simulink model "simulation"  (R2023b)
settings: Solver=VariableStepAuto  StartTime=0.0  StopTime=1.2  RelTol=1e-3
values from neighbouring files (symbols this model uses):
  J = [0 -1; 1 0]    [SafetyFilterSystemDPC.m]    (also in init.m)
undefined symbols (not defined in the file or in its folder): ctrl, DiscIntNeverNeededParam, fdesignblkfcn, gcbh, grid, infinite_bus, load1, overcurr_ctrl, pll, pq_ctrl, pv, sim, soa
libraries: spsabctodq0Lib x8, eeGeneralControl x6, spsControlledVoltageSourceLib x6, eeDiscretePi x5, dsparch4 x4, spsBreakerLib x3, spsThreePhaseSeriesRLCBranchLib x3, spsdq0toabcLib x2, spsThreePhaseBreakerLib x2, simulink x1, spsGroundLib x1, spsThreePhaseVIMeasurementLib x1
settings Model: SimulationMode=accelerator  Creator=ma1155716  LastModifiedBy=ma1155716

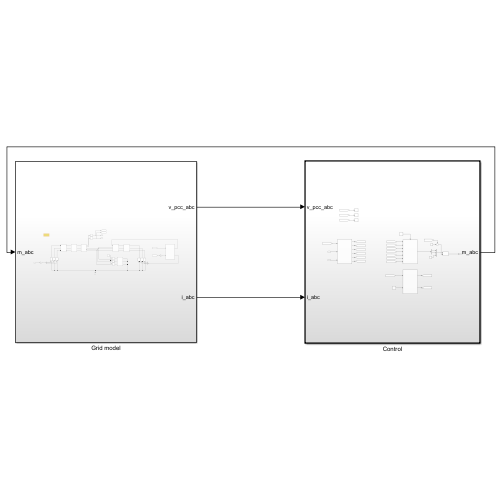
[thumbnail: Simulink's stored preview of the top-level diagram]
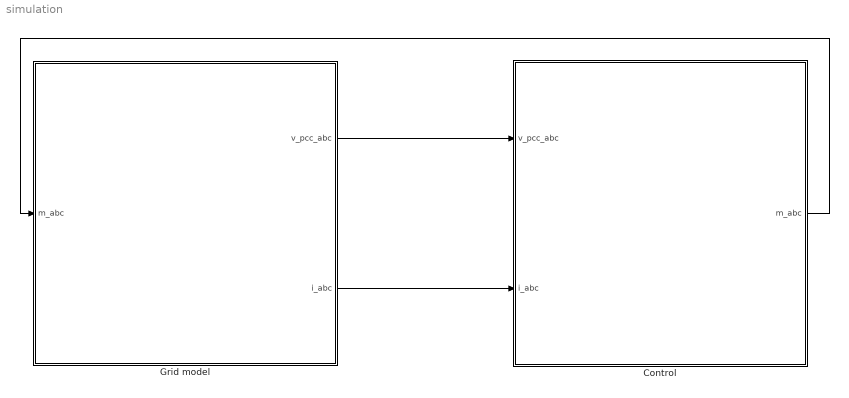
== system simulation ==
  Control : Subsystem  TreatAsAtomicUnit=on
  Grid model : Subsystem
  wires:
  Grid model/1(v_pcc_abc) -> Control/1(v_pcc_abc)
  Control/1(m_abc) -> Grid model/1(m_abc)
  Grid model/2(i_abc) -> Control/2(i_abc)

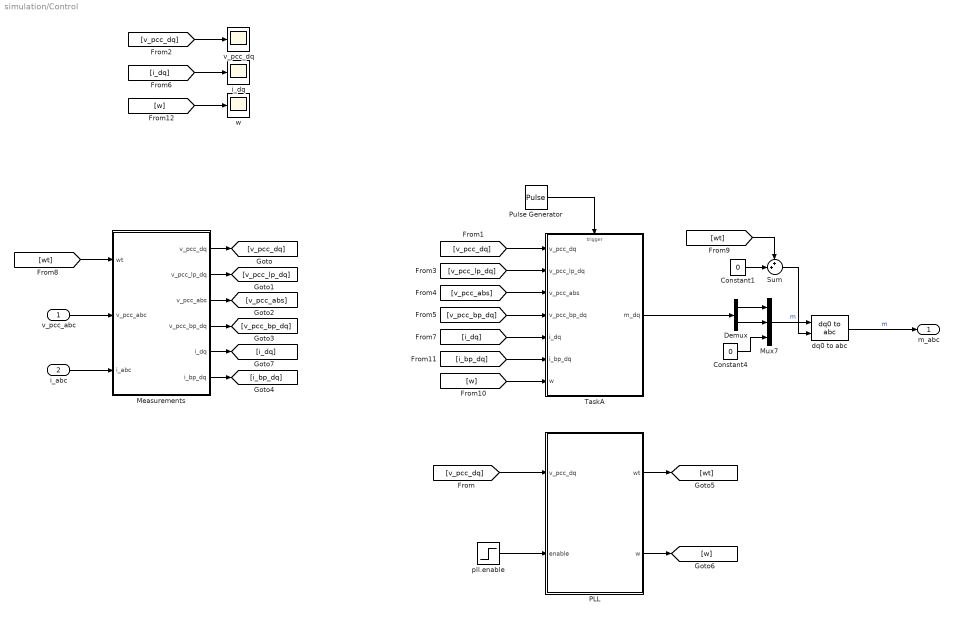
== system simulation/Control ==
  v_pcc_abc : Inport
  i_abc : Inport  Port=2
  Constant1 : Constant  Value=0
  Constant4 : Constant  Value=0
  Demux : Demux  Outputs=2
  Measurements : Subsystem
  Mux7 : Mux  Inputs=3
  PLL : Subsystem
  Pulse Generator : DiscretePulseGenerator  PulseType=Time based  Period=ctrl.ts  PulseWidth=50
  Sum : Sum  Inputs=++|
  TaskA : Subsystem
  dq0 to abc : spsdq0toabcLib/dq0 to abc  Alignment=Aligned with phase A axis
  i_dq : Scope
  "pll.enable " : Step  Time=pll.enable
  v_pcc_dq : Scope
  w : Scope
  m_abc : Outport  InitialOutput=[1;0;0]
  wires:
  v_pcc_abc/1 -> Measurements/2(v_pcc_abc)
  i_abc/1 -> Measurements/3(i_abc)
  Pulse Generator/1 -> TaskA/Trigger
  Demux/1 -> Mux7/1
  Constant4/1 -> Mux7/3
  Demux/2 -> Mux7/2
  TaskA/1(m_dq) -> Demux/1
  Mux7/1 -> dq0 to abc/1  "m"
  dq0 to abc/1 -> m_abc/1  "m"
  Sum/1 -> dq0 to abc/2
  Constant1/1 -> Sum/2
  Measurements/1(v_pcc_dq) -> [v_pcc_dq]
  [v_pcc_dq] -> PLL/1(v_pcc_dq)
  [v_pcc_dq] -> TaskA/1(v_pcc_dq)
  Measurements/2(v_pcc_lp_dq) -> [v_pcc_lp_dq]
  [v_pcc_lp_dq] -> TaskA/2(v_pcc_lp_dq)
  [v_pcc_dq] -> v_pcc_dq/1
  Measurements/3(v_pcc_abs) -> [v_pcc_abs]
  Measurements/4(v_pcc_bp_dq) -> [v_pcc_bp_dq]
  [v_pcc_abs] -> TaskA/3(v_pcc_abs)
  [v_pcc_bp_dq] -> TaskA/4(v_pcc_bp_dq)
  Measurements/6(i_bp_dq) -> [i_bp_dq]
  [i_dq] -> i_dq/1
  [i_dq] -> TaskA/5(i_dq)
  PLL/1(wt) -> [wt]
  [wt] -> Measurements/1(wt)
  [wt] -> Sum/1
  PLL/2(w) -> [w]
  [w] -> TaskA/7(w)
  Measurements/5(i_dq) -> [i_dq]
  [i_bp_dq] -> TaskA/6(i_bp_dq)
  "pll.enable "/1 -> PLL/2(enable)
  [w] -> w/1

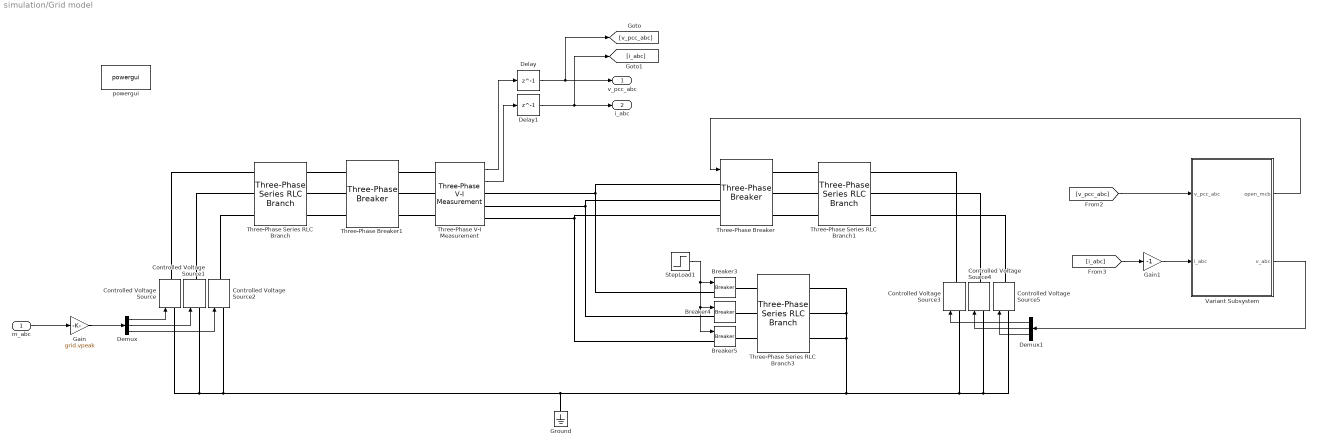
== system simulation/Grid model ==
  m_abc : Inport
  Breaker3 : spsBreakerLib/Breaker  InitialState=0  SwitchingTimes="[1/60  5/60]"  External=on  BreakerResistance=0.01  SnubberResistance=1e6  SnubberCapacitance=inf  Measurements=None  MoreParameters=on  NoBreakLoop=off
  Breaker4 : spsBreakerLib/Breaker  InitialState=0  SwitchingTimes="[1/60  5/60]"  External=on  BreakerResistance=0.01  SnubberResistance=1e6  SnubberCapacitance=inf  Measurements=None  MoreParameters=on  NoBreakLoop=off
  Breaker5 : spsBreakerLib/Breaker  InitialState=0  SwitchingTimes="[1/60  5/60]"  External=on  BreakerResistance=0.01  SnubberResistance=1e6  SnubberCapacitance=inf  Measurements=None  MoreParameters=on  NoBreakLoop=off
  Controlled Voltage Source{,1..5} (6 alike) : spsControlledVoltageSourceLib/Controlled Voltage Source  Initialize=on  Source_Type=AC  Amplitude=0  Phase=0  Frequency=0  Measurements=None
  Delay : Delay  DelayLength=1  InitialCondition=0  SampleTime=sim.ts
  Delay1 : Delay  DelayLength=1  InitialCondition=0  SampleTime=sim.ts
  Demux : Demux  Outputs=3
  Demux1 : Demux  Outputs=3
  Gain : Gain  Gain=grid.vpeak
  Gain1 : Gain  Gain=-1
  Ground : spsGroundLib/Ground  LConnTagsString=a
  StepLoad1 : Step  Time=load1.stepTime  SampleTime=0
  Three-Phase Series RLC Branch : spsThreePhaseSeriesRLCBranchLib/Three-Phase Series RLC Branch  LConnTagsString=A|B|C  RConnTagsString=A|B|C  BranchType=RL  Resistance=grid.r1_si  Inductance=grid.l1_si  Capacitance=1e-6  Measurements=None
  Three-Phase Series RLC Branch1 : spsThreePhaseSeriesRLCBranchLib/Three-Phase Series RLC Branch  LConnTagsString=A|B|C  RConnTagsString=A|B|C  BranchType=RL  Resistance=grid.r2_si  Inductance=grid.l2_si  Capacitance=1e-6  Measurements=None
  Three-Phase Series RLC Branch3 : spsThreePhaseSeriesRLCBranchLib/Three-Phase Series RLC Branch  LConnTagsString=A|B|C  RConnTagsString=A|B|C  BranchType=RL  Resistance=load1.r_si  Inductance=load1.l_si  Capacitance=1e-6  Measurements=None
  Three-Phase V-I Measurement : spsThreePhaseVIMeasurementLib/Three-Phase V-I Measurement  VoltageMeasurement=phase-to-ground  SetLabelV=off  LabelV=Vabc  Vpu=off  VpuLL=off  CurrentMeasurement=yes  SetLabelI=off  LabelI=Iabc  Ipu=off  Pbase=100e6  Vbase=500e3  OutputType=Complex  PhasorSimulation=off  PSBequivalent=0
  Three-Phase Breaker : spsThreePhaseBreakerLib/Three-Phase Breaker  InitialState=open  SwitchA=on  SwitchB=on  SwitchC=on  SwitchTimes=[grid.close_mcb2]  External=on  BreakerResistance=0.01  SnubberResistance=1e6  SnubberCapacitance=inf  Measurements=None
  Three-Phase Breaker1 : spsThreePhaseBreakerLib/Three-Phase Breaker  InitialState=open  SwitchA=on  SwitchB=on  SwitchC=on  SwitchTimes=[0]  External=off  BreakerResistance=0.01  SnubberResistance=1e6  SnubberCapacitance=inf  Measurements=None
  Variant Subsystem : Subsystem  Variant=on
  powergui : spspowerguiLib/powergui  Priority=1  SimulationMode=Discrete  SampleTime=sim.ts  frequency=60  Iterations=50  frequencyindice=0  Pbase=100e6  ErrMax=1e-4  UnitsV=kV  UnitsW=MW  buscounter=0  FunctionMessages=off  echomessages=off  EnableUseOfTLC=off  CurrentSourceSwitches=off  DisableSnubberDevices=off  DisableRonSwitches=off  DisableVfSwitches=off  DisplayEquations=off  AutomaticDiscreteSolvers=off  SolverType=Tustin/Backward Euler (TBE)  Interpol=off  ExternalGateDelay=off  methode=off  Ts=100  x0status=blocks  SPID=on  SwTol=0  HookPort=off  NonlinearTolerance=1e-4  nMaxIteration=100  ContinueOnMaxIteration=off  RestoreLinks=warning  ResistiveCurrentMeasurement=off  Frange=[0:2:500]  Ylog=off  Xlog=on  ShowGrid=off  save=off  variable=ZData  structure=0  ZoomFFT=off  StartTime=0.0  cycles=1  DisplayStyle=1  fundamental=60  FreqAxis=off  MaxFrequency=1000  frequencyindicesteady=1  RmsSteady=1  display=off
  v_pcc_abc : Outport
  i_abc : Outport  Port=2
  wires:
  m_abc/1 -> Gain/1
  Demux/1 -> Controlled Voltage Source/1
  Demux/2 -> Controlled Voltage Source1/1
  Demux/3 -> Controlled Voltage Source2/1
  Demux1/3 -> Controlled Voltage Source5/1
  Demux1/1 -> Controlled Voltage Source3/1
  Three-Phase V-I Measurement/1 -> Delay/1
  Three-Phase V-I Measurement/2 -> Delay1/1
  Gain/1 -> Demux/1
  Demux1/2 -> Controlled Voltage Source4/1
  StepLoad1/1 -> Breaker5/1, Breaker4/1, Breaker3/1
  Delay1/1 -> [i_abc], i_abc/1
  Delay/1 -> [v_pcc_abc], v_pcc_abc/1
  [v_pcc_abc] -> Variant Subsystem/1(v_pcc_abc)
  [i_abc] -> Gain1/1
  Variant Subsystem/2(v_abc) -> Demux1/1
  Gain1/1 -> Variant Subsystem/2(i_abc)
  Variant Subsystem/1(open_mcb) -> Three-Phase Breaker/1
  connections:
  Three-Phase Series RLC Branch/LConn1 -- Controlled Voltage Source/RConn1
  Three-Phase Series RLC Branch/LConn2 -- Controlled Voltage Source1/RConn1
  Controlled Voltage Source2/RConn1 -- Three-Phase Series RLC Branch/LConn3
  Three-Phase Series RLC Branch/RConn1 -- Three-Phase Breaker1/LConn1
  Three-Phase Series RLC Branch/RConn2 -- Three-Phase Breaker1/LConn2
  Three-Phase Series RLC Branch/RConn3 -- Three-Phase Breaker1/LConn3
  Breaker3/LConn1 -- Three-Phase Breaker/LConn1 -- Three-Phase V-I Measurement/RConn1
  Breaker4/LConn1 -- Three-Phase V-I Measurement/RConn2 -- Three-Phase Breaker/LConn2
  Breaker5/LConn1 -- Three-Phase Breaker/LConn3 -- Three-Phase V-I Measurement/RConn3
  Controlled Voltage Source3/RConn1 -- Three-Phase Series RLC Branch1/RConn1
  Controlled Voltage Source4/RConn1 -- Three-Phase Series RLC Branch1/RConn2
  Controlled Voltage Source5/RConn1 -- Three-Phase Series RLC Branch1/RConn3
  Ground/LConn1 -- Controlled Voltage Source3/LConn1 -- Controlled Voltage Source5/LConn1 -- Controlled Voltage Source4/LConn1 -- Three-Phase Series RLC Branch3/RConn3 -- Three-Phase Series RLC Branch3/RConn2 -- Three-Phase Series RLC Branch3/RConn1 -- Controlled Voltage Source2/LConn1 -- Controlled Voltage Source1/LConn1 -- Controlled Voltage Source/LConn1
  Breaker4/RConn1 -- Three-Phase Series RLC Branch3/LConn2
  Breaker5/RConn1 -- Three-Phase Series RLC Branch3/LConn3
  Three-Phase Series RLC Branch3/LConn1 -- Breaker3/RConn1
  Three-Phase Series RLC Branch1/LConn1 -- Three-Phase Breaker/RConn1
  Three-Phase Series RLC Branch1/LConn2 -- Three-Phase Breaker/RConn2
  Three-Phase Series RLC Branch1/LConn3 -- Three-Phase Breaker/RConn3
  Three-Phase Breaker1/RConn1 -- Three-Phase V-I Measurement/LConn1
  Three-Phase Breaker1/RConn2 -- Three-Phase V-I Measurement/LConn2
  Three-Phase Breaker1/RConn3 -- Three-Phase V-I Measurement/LConn3

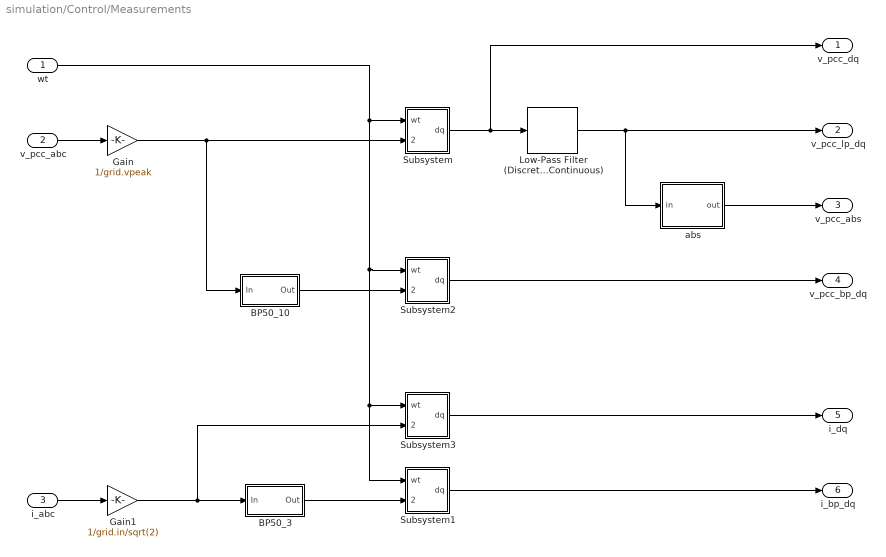
== system simulation/Control/Measurements ==
  wt : Inport
  v_pcc_abc : Inport  Port=2
  i_abc : Inport  Port=3
  BP50_10 : Subsystem  DialogController=fdesignblkfcn  InitFcn=fdesignblkfcn(gcbh, {'InitFcn'});  mask(Bandpass Filter){}
      mask help: dsp:DSPFilterDesignBlockDialog:BandpassFdesign_MaskDesc
      settings: CopyFcn=fdesignblkfcn(gcbh, {'CopyFcn'});
      mask Help: helpview(mapfilelocation('dsp'), 'dspbandpassfilter');
      mask Display: disp('Bandpass');
  BP50_3 : Subsystem  DialogController=fdesignblkfcn  InitFcn=fdesignblkfcn(gcbh, {'InitFcn'});  mask(Bandpass Filter){}
      mask help: dsp:DSPFilterDesignBlockDialog:BandpassFdesign_MaskDesc
      settings: CopyFcn=fdesignblkfcn(gcbh, {'CopyFcn'});
      mask Help: helpview(mapfilelocation('dsp'), 'dspbandpassfilter');
      mask Display: disp('Bandpass');
  Gain : Gain  Gain=1/grid.vpeak
  Gain1 : Gain  Gain=1/grid.in/sqrt(2)
  Low-Pass Filter (Discrete or Continuous) : eeGeneralControl/Low-Pass Filter (Discrete or Continuous)  K=1  T=1/grid.w0*10  B=inf  A=-inf  init_option=Inherited from block input  x0=0  Ts=-1
  Subsystem : Subsystem
  Subsystem1 : Subsystem
  Subsystem2 : Subsystem
  Subsystem3 : Subsystem
  abs : Subsystem
  v_pcc_dq : Outport
  v_pcc_lp_dq : Outport  Port=2
  v_pcc_abs : Outport  Port=3
  v_pcc_bp_dq : Outport  Port=4
  i_dq : Outport  Port=5
  i_bp_dq : Outport  Port=6
  wires:
  v_pcc_abc/1 -> Gain/1
  Subsystem/1(dq) -> v_pcc_dq/1, Low-Pass Filter (Discrete or Continuous)/1
  Gain/1 -> BP50_10/1(In), Subsystem/2(abc)
  i_abc/1 -> Gain1/1
  BP50_3/1(Out) -> Subsystem1/2(abc)
  Subsystem1/1(dq) -> i_bp_dq/1
  Gain1/1 -> Subsystem3/2(abc), BP50_3/1(In)
  Low-Pass Filter (Discrete or Continuous)/1 -> abs/1(in), v_pcc_lp_dq/1
  BP50_10/1(Out) -> Subsystem2/2(abc)
  Subsystem2/1(dq) -> v_pcc_bp_dq/1
  wt/1 -> Subsystem2/1(wt), Subsystem3/1(wt), Subsystem1/1(wt), Subsystem/1(wt)
  Subsystem3/1(dq) -> i_dq/1
  abs/1(out) -> v_pcc_abs/1

== system simulation/Control/PLL ==
  v_pcc_dq : Inport
  enable : Inport  Port=2
  Complex to Magnitude-Angle : ComplexToMagnitudeAngle
  Constant : Constant  Value=0
  Constant1 : Constant  Value=0
  Demux6 : Demux  Outputs=2
  Discrete PI Controller : eeDiscretePi/Discrete PI Controller  Kp=pll.kp  Ki=pll.ki  Kaw=1  x0=pll.init_w  Ts=-1
      settings: LibrarySourceBlock=ee_sl_lib/General Control/Discrete PI Controller
  Discrete-Time Integrator : DiscreteIntegrator  gainval=grid.w0  SampleTime=-1  ICPrevOutput=DiscIntNeverNeededParam  ICPrevScaledInput=DiscIntNeverNeededParam
  NOT1 : Logic  Operator=NOT  IconShape=distinctive  AllPortsSameDT=off  OutDataTypeStr=boolean
  Real-Imag to Complex : RealImagToComplex
  Switch : Switch  Criteria=u2 > Threshold  SaturateOnIntegerOverflow=off  InputSameDT=off
  Terminator7 : Terminator
  wt : Outport
  w : Outport  Port=2
  wires:
  v_pcc_dq/1 -> Demux6/1  "v_pcc_dq"
  Complex to Magnitude-Angle/1 -> Terminator7/1
  Demux6/2 -> Real-Imag to Complex/2  "v_pll_q"
  Complex to Magnitude-Angle/2 -> Switch/3  "theta_v_pll"
  Real-Imag to Complex/1 -> Complex to Magnitude-Angle/1
  Demux6/1 -> Real-Imag to Complex/1  "v_pll_d"
  Constant/1 -> Discrete PI Controller/2
  Discrete PI Controller/1 -> w/1, Discrete-Time Integrator/1
  Discrete-Time Integrator/1 -> wt/1
  NOT1/1 -> Switch/2, Discrete PI Controller/3
  enable/1 -> NOT1/1
  Switch/1 -> Discrete PI Controller/1
  Constant1/1 -> Switch/1

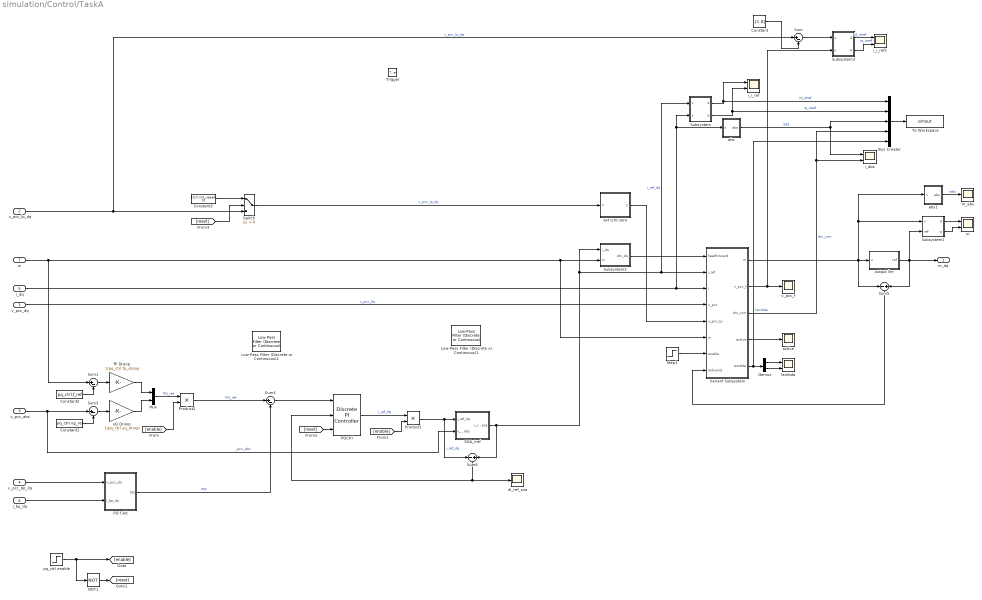
== system simulation/Control/TaskA ==
  v_pcc_dq : Inport
  v_pcc_lp_dq : Inport  Port=2
  v_pcc_abs : Inport  Port=3
  v_pcc_bp_dq : Inport  Port=4
  i_dq : Inport  Port=5
  i_bp_dq : Inport  Port=6
  w : Inport  Port=7
  Trigger : TriggerPort  VariantControl=(inherit)
  Bus Creator : BusCreator  Inputs=5
  Constant : Constant  Value=[1 0]
  Constant1 : Constant  Value=pq_ctrl.vg_ref
  Constant2 : Constant  Value=pq_ctrl.f_ref
  Constant3 : Constant  Value=[ctrl.init_vpeak; 0]
  Demux : Demux  Outputs=2
  Low-Pass Filter (Discrete or Continuous)1 : eeGeneralControl/Low-Pass Filter (Discrete or Continuous)  K=1  T=1e-3  B=inf  A=-inf  init_option=Inherited from block input  x0=0  Ts=-1
  Low-Pass Filter (Discrete or Continuous)2 : eeGeneralControl/Low-Pass Filter (Discrete or Continuous)  K=1  T=1e-2  B=inf  A=-inf  init_option=Inherited from block input  x0=0  Ts=-1
  Mux : Mux  Inputs=2
  NOT1 : Logic  Operator=NOT  IconShape=distinctive  AllPortsSameDT=off  OutDataTypeStr=boolean
  PQ Calc : Subsystem
  PQCtrl : eeDiscretePi/Discrete PI Controller  Kp=pq_ctrl.kp  Ki=pq_ctrl.ki  Kaw=100  x0=0  Ts=-1
      settings: LibrarySourceBlock=ee_sl_lib/General Control/Discrete PI Controller
  Product1 : Product
  Product2 : Product
  SOA_iref : Subsystem
  Step1 : Step  Time=overcurr_ctrl.enableTime
  Subsystem : Subsystem
  Subsystem1 : Subsystem
  Subsystem2 : Subsystem
  Subsystem3 : Subsystem
  Sum{,1,3..4} (4 alike) : Sum  Inputs=|+-
  Sum5 : Sum  Inputs=-|+
  Sum6 : Sum  Inputs=-|+
  Switch : Switch  Criteria=u2 > Threshold  SaturateOnIntegerOverflow=off  InputSameDT=off
  To Workspace : ToWorkspace  VariableName=simout  SaveFormat=Timeseries  SampleTime=-1
  Variant Subsystem : Subsystem  Variant=on
  abs : Subsystem
  abs1 : Subsystem
  active : Scope
  di_ref_soa : Scope
  fP Droop : Gain  Gain=1/pq_ctrl.fp_droop
  i_abs : Scope  NumInputPorts=2
  i_i_ref : Scope  NumInputPorts=2
  i_i_ref1 : Scope  NumInputPorts=2
  lambda : Scope  NumInputPorts=2
  m : Scope  NumInputPorts=2
  m_abs : Scope
  output lim : Subsystem
  pq_ctrl.enable : Step  Time=pq_ctrl.enable
  set q to zero : Subsystem
  uQ Droop : Gain  Gain=1/pq_ctrl.uq_droop
  v_pcc_f : Scope
  m_dq : Outport  InitialOutput=[ctrl.init_vpeak 0]
  wires:
  SOA_iref/1(i_ref_dq_soa) -> Subsystem/1(x), Variant Subsystem/2(i_ref), Subsystem2/1(i_dq), Sum6/2  "i_ref_dq"
  w/1 -> Subsystem2/2(w), Variant Subsystem/6(w), Sum1/1
  Switch/1 -> set q to zero/1(x)  "v_pcc_lp_dq"
  Variant Subsystem/1(m) -> abs1/1(x), Subsystem1/1(x), output lim/1(x), Sum5/1
  v_pcc_dq/1 -> Variant Subsystem/4(v_pcc)  "v_pcc_dq"
  i_dq/1 -> Subsystem/2(y), abs/1(x), Variant Subsystem/3(i)
  Sum1/1 -> fP Droop/1
  Constant1/1 -> Sum3/2
  Sum3/1 -> uQ Droop/1
  fP Droop/1 -> Mux/1
  uQ Droop/1 -> Mux/2
  Product2/1 -> Sum4/1  "PQ_ref"
  Sum4/1 -> PQCtrl/1
  Sum6/1 -> di_ref_soa/1, PQCtrl/2
  v_pcc_abs/1 -> SOA_iref/2(v_pcc_abs), Sum3/1  "_pcc_abs"
  v_pcc_bp_dq/1 -> PQ Calc/1(v_pcc_dq)
  Mux/1 -> Product2/1  "PQ_ref"
  PQCtrl/1 -> Product1/1  "i_ref_dq"
  i_bp_dq/1 -> PQ Calc/2(i_bp_dq)
  output lim/1(ref) -> Subsystem1/2(ref), m_dq/1, Sum5/2
  pq_ctrl.enable/1 -> NOT1/1, [enable]
  [enable] -> Product2/2
  [enable] -> Product1/2
  NOT1/1 -> [reset]
  [reset] -> PQCtrl/3
  PQ Calc/1(PQ) -> Sum4/2  "PW"
  Product1/1 -> SOA_iref/1(i_ref_dq), Sum6/1  "i_ref_dq"
  abs/1(abs) -> Bus Creator/3, i_abs/1  "iabs"
  Constant2/1 -> Sum1/2
  Subsystem/1(d) -> i_i_ref/1, Bus Creator/1  "id_idref"
  Subsystem/2(q) -> i_i_ref/2, Bus Creator/2  "iq_iqref"
  Subsystem1/1(d) -> m/1
  Subsystem1/2(q) -> m/2
  Sum5/1 -> Variant Subsystem/8(antiwind)
  Step1/1 -> Variant Subsystem/7(enable)
  Variant Subsystem/4(active) -> active/1
  Bus Creator/1 -> To Workspace/1
  abs1/1(abs) -> m_abs/1  "iabs"
  Subsystem2/1(dm_dq) -> Variant Subsystem/1(feedforward)
  [reset] -> Switch/2
  Constant3/1 -> Switch/1
  v_pcc_lp_dq/1 -> Sum/1, Switch/3  "v_pcc_lp_dq"
  Demux/2 -> lambda/2
  Demux/1 -> lambda/1
  Variant Subsystem/5(lambda) -> Bus Creator/5, Demux/1  "lambda"
  Variant Subsystem/2(v_pcc_f) -> Subsystem3/2(y), v_pcc_f/1
  Variant Subsystem/3(dm_corr) -> i_abs/2, Bus Creator/4  "dm_corr"
  set q to zero/1(y) -> Variant Subsystem/5(v_pcc_lp)
  Subsystem3/1(d) -> i_i_ref1/1  "id_idref"
  Subsystem3/2(q) -> i_i_ref1/2  "iq_iqref"
  Sum/1 -> Subsystem3/1(x)
  Constant/1 -> Sum/2

== system simulation/Grid model/Variant Subsystem ==
  note: 1) Add Subsystem or Model blocks as valid variant choices.
      | 2) You cannot connect blocks at this level. At simulation, connectivity is automatically
      | determined, based on the active variant and port name matching.
  v_pcc_abc : Inport
  i_abc : Inport  Port=2
  infinite_bus : Subsystem  VariantControl=grid.sel==0
  open : Subsystem  VariantControl=grid.sel==2
  static_converter : Subsystem  VariantControl=grid.sel==1
  open_mcb : Outport
  v_abc : Outport  Port=2

== system simulation/Control/Measurements/BP50_10 ==
  In : Inport
  Generated Filter Block : dsparch4/Biquad Filter  Tag=BlockMethodSubSystem  FilterSource=Dialog parameters  CoeffSource=Specify via dialog  FilterObject=BQF  IIRFiltStruct=Direct form II  BiQuadCoeffs=[2 0 -2 1 -1.99996903213533184 0.99996913076816718]  ScaleValues=[4.98592317955378183e-08;154.7819266430281]  IC=0  ICnum=0  ICden=0  a0Flag=Warning  optimizeScaleValues=off  ScaleValueMode=Specify via input port (g)  roundingMode=Floor  overflowMode=off  scaleValueFracLength=14  denProdOutputFracLength=30  denAccumFracLength=30  secondMemoryFracLength=15
  Out : Outport  VectorParamsAs1DForOutWhenUnconnected=off
  wires:
  In/1 -> Generated Filter Block/1
  Generated Filter Block/1 -> Out/1

== system simulation/Control/Measurements/BP50_3 ==
  In : Inport
  Generated Filter Block : dsparch4/Biquad Filter  Tag=BlockMethodSubSystem  FilterSource=Dialog parameters  CoeffSource=Specify via dialog  FilterObject=BQF  IIRFiltStruct=Direct form II  BiQuadCoeffs=[2 0 -2 1 -1.99996903213533184 0.99996913076816718]  ScaleValues=[4.98592317955378183e-08;154.7819266430281]  IC=0  ICnum=0  ICden=0  a0Flag=Warning  optimizeScaleValues=off  ScaleValueMode=Specify via input port (g)  roundingMode=Floor  overflowMode=off  scaleValueFracLength=14  denProdOutputFracLength=30  denAccumFracLength=30  secondMemoryFracLength=15
  Out : Outport  VectorParamsAs1DForOutWhenUnconnected=off
  wires:
  In/1 -> Generated Filter Block/1
  Generated Filter Block/1 -> Out/1

== system simulation/Control/Measurements/Subsystem ==
  wt : Inport
  abc : Inport  Port=2
  Demux6 : Demux  Outputs=3
  Mux : Mux  Inputs=2
  Terminator7 : Terminator
  abc_dq_1 : spsabctodq0Lib/abc to dq0  Alignment=Aligned with phase A axis
  dq : Outport
  wires:
  Demux6/3 -> Terminator7/1
  Demux6/2 -> Mux/2  "v_pll_q"
  wt/1 -> abc_dq_1/2
  Mux/1 -> dq/1
  Demux6/1 -> Mux/1  "v_pll_d"
  abc/1 -> abc_dq_1/1
  abc_dq_1/1 -> Demux6/1

== system simulation/Control/Measurements/Subsystem1 ==
  wt : Inport
  abc : Inport  Port=2
  Demux6 : Demux  Outputs=3
  Mux : Mux  Inputs=2
  Terminator7 : Terminator
  abc_dq_1 : spsabctodq0Lib/abc to dq0  Alignment=Aligned with phase A axis
  dq : Outport
  wires:
  Demux6/3 -> Terminator7/1
  Demux6/2 -> Mux/2  "v_pll_q"
  wt/1 -> abc_dq_1/2
  Mux/1 -> dq/1
  Demux6/1 -> Mux/1  "v_pll_d"
  abc/1 -> abc_dq_1/1
  abc_dq_1/1 -> Demux6/1

== system simulation/Control/Measurements/Subsystem2 ==
  wt : Inport
  abc : Inport  Port=2
  Demux6 : Demux  Outputs=3
  Mux : Mux  Inputs=2
  Terminator7 : Terminator
  abc_dq_1 : spsabctodq0Lib/abc to dq0  Alignment=Aligned with phase A axis
  dq : Outport
  wires:
  Demux6/3 -> Terminator7/1
  Demux6/2 -> Mux/2  "v_pll_q"
  wt/1 -> abc_dq_1/2
  Mux/1 -> dq/1
  Demux6/1 -> Mux/1  "v_pll_d"
  abc/1 -> abc_dq_1/1
  abc_dq_1/1 -> Demux6/1

== system simulation/Control/Measurements/Subsystem3 ==
  wt : Inport
  abc : Inport  Port=2
  Demux6 : Demux  Outputs=3
  Mux : Mux  Inputs=2
  Terminator7 : Terminator
  abc_dq_1 : spsabctodq0Lib/abc to dq0  Alignment=Aligned with phase A axis
  dq : Outport
  wires:
  Demux6/3 -> Terminator7/1
  Demux6/2 -> Mux/2  "v_pll_q"
  wt/1 -> abc_dq_1/2
  Mux/1 -> dq/1
  Demux6/1 -> Mux/1  "v_pll_d"
  abc/1 -> abc_dq_1/1
  abc_dq_1/1 -> Demux6/1

== system simulation/Control/Measurements/abs ==
  in : Inport
  Complex to Magnitude-Angle1 : ComplexToMagnitudeAngle
  Demux : Demux  Outputs=2
  Real-Imag to Complex1 : RealImagToComplex
  Terminator : Terminator
  out : Outport
  wires:
  Complex to Magnitude-Angle1/1 -> out/1  "V_pcc_meas"
  Demux/2 -> Real-Imag to Complex1/2
  Demux/1 -> Real-Imag to Complex1/1
  Complex to Magnitude-Angle1/2 -> Terminator/1
  Real-Imag to Complex1/1 -> Complex to Magnitude-Angle1/1
  in/1 -> Demux/1

== system simulation/Control/TaskA/PQ Calc ==
  v_pcc_dq : Inport
  i_bp_dq : Inport  Port=2
  Gain2 : Gain  Gain=J  Multiplication=Matrix(K*u) (u vector)
  Low-Pass Filter (Discrete or Continuous) : eeGeneralControl/Low-Pass Filter (Discrete or Continuous)  K=1  T=1/grid.w0  B=inf  A=-inf  init_option=Inherited from block input  x0=0  Ts=-1
  Mux : Mux  Inputs=2
  Product1 : Product  Multiplication=Matrix(*)
  Product2 : Product  Multiplication=Matrix(*)
  Transpose : Math  Operator=transpose
  Transpose1 : Math  Operator=transpose
  PQ : Outport
  wires:
  Gain2/1 -> Transpose1/1
  v_pcc_dq/1 -> Transpose/1, Gain2/1
  i_bp_dq/1 -> Product1/2, Product2/2
  Product1/1 -> Mux/1
  Product2/1 -> Mux/2
  Transpose1/1 -> Product2/1
  Transpose/1 -> Product1/1
  Low-Pass Filter (Discrete or Continuous)/1 -> PQ/1
  Mux/1 -> Low-Pass Filter (Discrete or Continuous)/1

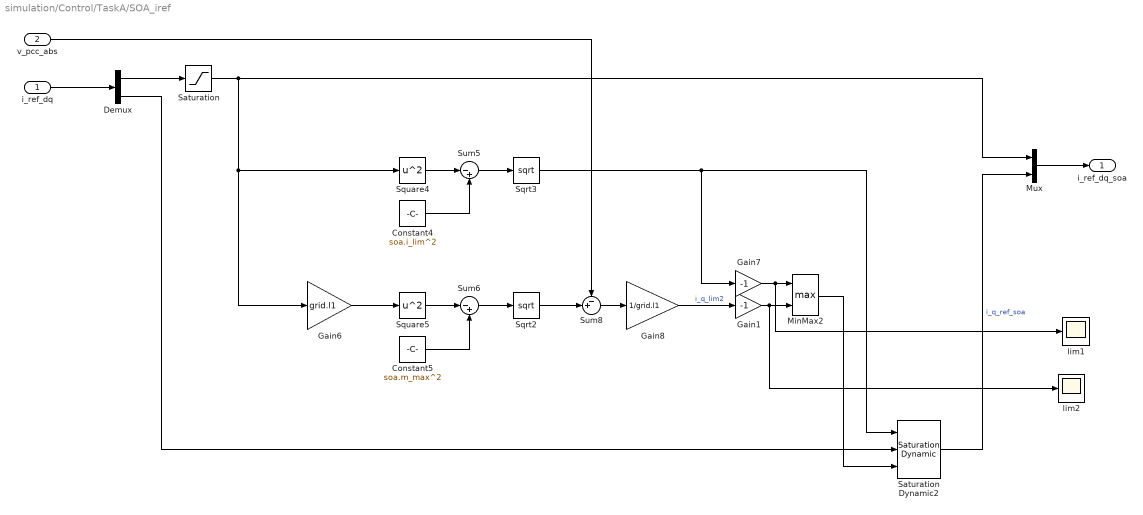
== system simulation/Control/TaskA/SOA_iref ==
  i_ref_dq : Inport
  v_pcc_abs : Inport  Port=2
  Constant4 : Constant  Value=soa.i_lim^2
  Constant5 : Constant  Value=soa.m_max^2
  Demux : Demux  Outputs=2
  Gain1 : Gain  Gain=-1
  Gain6 : Gain  Gain=grid.l1
  Gain7 : Gain  Gain=-1
  Gain8 : Gain  Gain=1/grid.l1
  MinMax2 : MinMax  Function=max  Inputs=2
  Mux : Mux  Inputs=2
  Saturation : Saturate  UpperLimit=soa.i_lim  LowerLimit=-soa.i_lim
  Saturation Dynamic2 : simulink/Discontinuities/Saturation Dynamic  OutMin=[]  OutMax=[]  OutDataTypeStr=Inherit: Same as second input  OutDataType=fixdt(1, 16)  OutScaling=2^-10  DoSatur=off
  Sqrt2 : Sqrt
  Sqrt3 : Sqrt
  Square4 : Math  Operator=square
  Square5 : Math  Operator=square
  Sum5 : Sum  Inputs=|-+
  Sum6 : Sum  Inputs=|-+
  Sum8 : Sum  Inputs=-+|
  lim1 : Scope
  lim2 : Scope
  i_ref_dq_soa : Outport
  wires:
  Saturation/1 -> Square4/1, Gain6/1, Mux/1
  Gain8/1 -> Gain1/1  "i_q_lim2"
  Sqrt3/1 -> Saturation Dynamic2/1, Gain7/1
  Gain6/1 -> Square5/1
  Demux/1 -> Saturation/1
  Square4/1 -> Sum5/1
  Sqrt2/1 -> Sum8/2
  Square5/1 -> Sum6/1
  Sum8/1 -> Gain8/1
  Constant5/1 -> Sum6/2
  Sum5/1 -> Sqrt3/1
  Demux/2 -> Saturation Dynamic2/2
  Constant4/1 -> Sum5/2
  MinMax2/1 -> Saturation Dynamic2/3
  i_ref_dq/1 -> Demux/1
  Gain7/1 -> lim1/1, MinMax2/1
  v_pcc_abs/1 -> Sum8/1
  Sum6/1 -> Sqrt2/1
  Saturation Dynamic2/1 -> Mux/2  "i_q_ref_soa"
  Mux/1 -> i_ref_dq_soa/1
  Gain1/1 -> lim2/1, MinMax2/2

== system simulation/Control/TaskA/Subsystem ==
  x : Inport
  y : Inport  Port=2
  Demux : Demux  Outputs=2
  Demux1 : Demux  Outputs=2
  Mux1 : Mux  Inputs=2
  Mux2 : Mux  Inputs=2
  d : Outport
  q : Outport  Port=2
  wires:
  Mux2/1 -> q/1
  y/1 -> Demux1/1
  Demux/2 -> Mux2/1
  Demux1/2 -> Mux2/2
  Demux/1 -> Mux1/1
  Demux1/1 -> Mux1/2
  Mux1/1 -> d/1
  x/1 -> Demux/1

== system simulation/Control/TaskA/Subsystem1 ==
  x : Inport
  ref : Inport  Port=2
  Demux : Demux  Outputs=2
  Demux1 : Demux  Outputs=2
  Mux1 : Mux  Inputs=2
  Mux2 : Mux  Inputs=2
  d : Outport
  q : Outport  Port=2
  wires:
  Mux2/1 -> q/1
  ref/1 -> Demux1/1
  Demux/2 -> Mux2/1
  Demux1/2 -> Mux2/2
  Demux/1 -> Mux1/1
  Demux1/1 -> Mux1/2
  Mux1/1 -> d/1
  x/1 -> Demux/1

== system simulation/Control/TaskA/Subsystem2 ==
  i_dq : Inport
  w : Inport  Port=2
  Gain : Gain  Gain=J  Multiplication=Matrix(K*u) (u vector)
  Gain1 : Gain  Gain=ctrl.l1
  Gain2 : Gain  Gain=ctrl.r1
  Product : Product
  Sum8 : Sum  Inputs=++|
  dm_dq : Outport
  wires:
  Gain1/1 -> Sum8/2
  Sum8/1 -> dm_dq/1  "dm_dq"
  Product/1 -> Gain/1
  Gain/1 -> Gain1/1  "dm_dq"
  w/1 -> Product/1
  i_dq/1 -> Gain2/1, Product/2
  Gain2/1 -> Sum8/1

== system simulation/Control/TaskA/Subsystem3 ==
  x : Inport
  y : Inport  Port=2
  Demux : Demux  Outputs=2
  Demux1 : Demux  Outputs=2
  Mux1 : Mux  Inputs=2
  Mux2 : Mux  Inputs=2
  d : Outport
  q : Outport  Port=2
  wires:
  Mux2/1 -> q/1
  y/1 -> Demux1/1
  Demux/2 -> Mux2/1
  Demux1/2 -> Mux2/2
  Demux/1 -> Mux1/1
  Demux1/1 -> Mux1/2
  Mux1/1 -> d/1
  x/1 -> Demux/1

== system simulation/Control/TaskA/Variant Subsystem ==
  feedforward : Inport
  i_ref : Inport  Port=2
  i : Inport  Port=3
  v_pcc : Inport  Port=4
  v_pcc_lp : Inport  Port=5
  w : Inport  Port=6
  enable : Inport  Port=7
  antiwind : Inport  Port=8
  current controller : Subsystem  VariantControl=overcurr_ctrl.sel==1
  passive : Subsystem  VariantControl=overcurr_ctrl.sel==0
  safety filter DPC : Subsystem  VariantControl=overcurr_ctrl.sel==2
  m : Outport
  v_pcc_f : Outport  Port=2
  dm_corr : Outport  Port=3
  active : Outport  Port=4
  lambda : Outport  Port=5

== system simulation/Control/TaskA/abs ==
  x : Inport
  Dot Product : DotProduct  OutDataTypeStr=Inherit: Inherit via internal rule
  Sqrt3 : Sqrt
  abs : Outport
  wires:
  Sqrt3/1 -> abs/1
  x/1 -> Dot Product/2, Dot Product/1
  Dot Product/1 -> Sqrt3/1

== system simulation/Control/TaskA/abs1 ==
  x : Inport
  Dot Product : DotProduct  OutDataTypeStr=Inherit: Inherit via internal rule
  Sqrt3 : Sqrt
  abs : Outport
  wires:
  Sqrt3/1 -> abs/1
  x/1 -> Dot Product/2, Dot Product/1
  Dot Product/1 -> Sqrt3/1

== system simulation/Control/TaskA/output lim ==
  x : Inport
  Constant6 : Constant  Value=soa.m_max
  Divide1 : Product  Inputs=*/
  Product4 : Product
  abs : Subsystem
  m_c_max<=u : Saturate  UpperLimit=inf  LowerLimit=soa.m_max
  ref : Outport
  wires:
  abs/1(abs) -> m_c_max<=u/1
  Constant6/1 -> Divide1/1
  Divide1/1 -> Product4/2  "a_s"
  m_c_max<=u/1 -> Divide1/2
  x/1 -> abs/1(x), Product4/1
  Product4/1 -> ref/1

== system simulation/Control/TaskA/set q to zero ==
  x : Inport
  Constant : Constant  Value=0
  Demux : Demux  Outputs=2
  Mux1 : Mux  Inputs=2
  Terminator : Terminator
  y : Outport
  wires:
  x/1 -> Demux/1
  Constant/1 -> Mux1/2
  Demux/1 -> Mux1/1
  Demux/2 -> Terminator/1
  Mux1/1 -> y/1  "PQ_ref"

== system simulation/Grid model/Variant Subsystem/infinite_bus ==
  v_pcc_abc : Inport
  i_abc : Inport  Port=2
  Constant : Constant
  Mux : Mux  Inputs=3
  Sine Wave : Sin  Amplitude=infinite_bus.vpeak  Frequency=infinite_bus.w  Phase=pi/2  SampleTime=0
  Sine Wave1 : Sin  Amplitude=infinite_bus.vpeak  Frequency=infinite_bus.w  Phase=pi/2-2*pi/3  SampleTime=0
  Sine Wave2 : Sin  Amplitude=infinite_bus.vpeak  Frequency=infinite_bus.w  Phase=pi/2+2*pi/3  SampleTime=0
  v_abc : Outport
  open_mcb : Outport  Port=2
  wires:
  Sine Wave/1 -> Mux/1
  Sine Wave1/1 -> Mux/2
  Sine Wave2/1 -> Mux/3
  Mux/1 -> v_abc/1
  Constant/1 -> open_mcb/1

== system simulation/Grid model/Variant Subsystem/open ==
  v_pcc_abc : Inport
  i_abc : Inport  Port=2
  Constant{1..4} (4 alike) : Constant  Value=0
  Mux : Mux  Inputs=3
  v_abc : Outport
  open_mcb : Outport  Port=2
  wires:
  Constant1/1 -> Mux/1
  Constant2/1 -> Mux/2
  Constant3/1 -> Mux/3
  Mux/1 -> v_abc/1
  Constant4/1 -> open_mcb/1

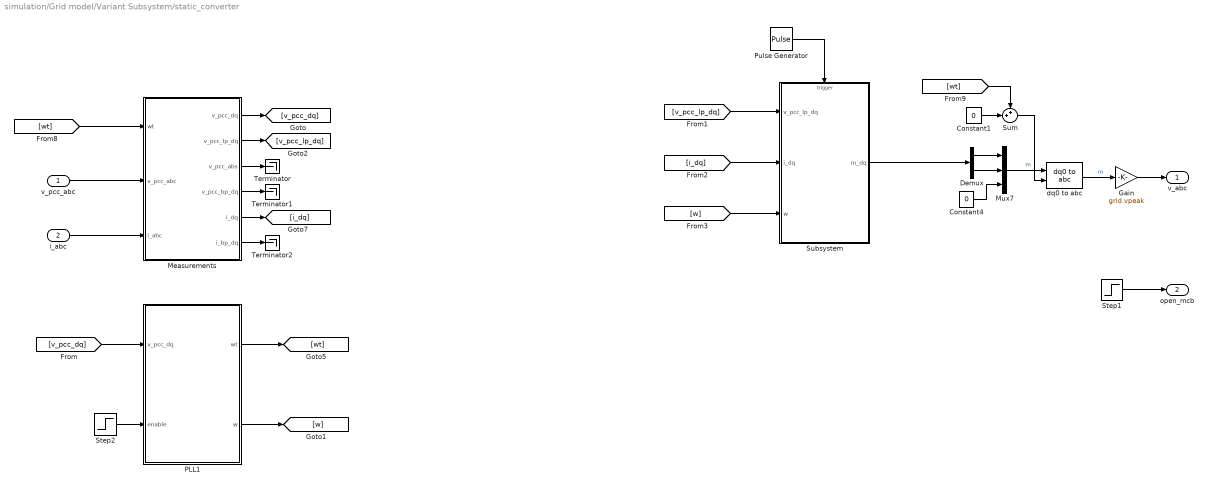
== system simulation/Grid model/Variant Subsystem/static_converter ==
  v_pcc_abc : Inport
  i_abc : Inport  Port=2
  Constant1 : Constant  Value=0
  Constant4 : Constant  Value=0
  Demux : Demux  Outputs=2
  Gain : Gain  Gain=grid.vpeak
  Measurements : Subsystem
  Mux7 : Mux  Inputs=3
  PLL1 : Subsystem
  Pulse Generator : DiscretePulseGenerator  PulseType=Time based  Period=ctrl.ts  PulseWidth=50
  Step1 : Step  Time=pv.open_mcp
  Step2 : Step  Time=pv.pll_enable
  Subsystem : Subsystem
  Sum : Sum  Inputs=++|
  Terminator : Terminator
  Terminator1 : Terminator
  Terminator2 : Terminator
  dq0 to abc : spsdq0toabcLib/dq0 to abc  Alignment=Aligned with phase A axis
  v_abc : Outport
  open_mcb : Outport  Port=2
  wires:
  v_pcc_abc/1 -> Measurements/2(v_pcc_abc)
  i_abc/1 -> Measurements/3(i_abc)
  [wt] -> Measurements/1(wt)
  PLL1/1(wt) -> [wt]
  Measurements/1(v_pcc_dq) -> [v_pcc_dq]
  [v_pcc_dq] -> PLL1/1(v_pcc_dq)
  PLL1/2(w) -> [w]
  Measurements/2(v_pcc_lp_dq) -> [v_pcc_lp_dq]
  Measurements/3(v_pcc_abs) -> Terminator/1
  Measurements/4(v_pcc_bp_dq) -> Terminator1/1
  Measurements/6(i_bp_dq) -> Terminator2/1
  Measurements/5(i_dq) -> [i_dq]
  Constant1/1 -> Sum/2
  Demux/2 -> Mux7/2
  Constant4/1 -> Mux7/3
  Mux7/1 -> dq0 to abc/1  "m"
  Demux/1 -> Mux7/1
  Sum/1 -> dq0 to abc/2
  dq0 to abc/1 -> Gain/1  "m"
  [wt] -> Sum/1
  Gain/1 -> v_abc/1
  Step2/1 -> PLL1/2(enable)
  Subsystem/1(m_dq) -> Demux/1
  [i_dq] -> Subsystem/2(i_dq)
  [w] -> Subsystem/3(w)
  Pulse Generator/1 -> Subsystem/Trigger
  [v_pcc_lp_dq] -> Subsystem/1(v_pcc_lp_dq)
  Step1/1 -> open_mcb/1

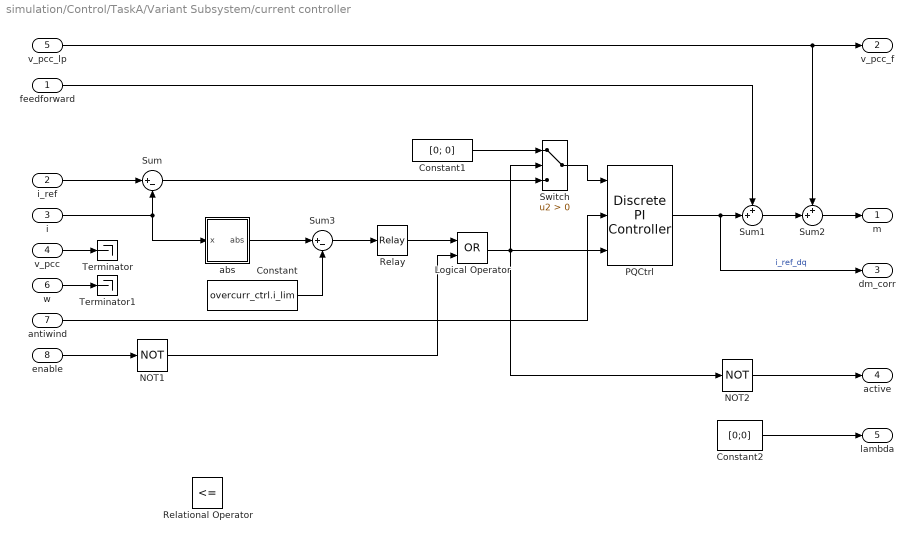
== system simulation/Control/TaskA/Variant Subsystem/current controller ==
  feedforward : Inport
  i_ref : Inport  Port=2
  i : Inport  Port=3
  v_pcc : Inport  Port=4
  v_pcc_lp : Inport  Port=5
  w : Inport  Port=6
  antiwind : Inport  Port=7
  enable : Inport  Port=8
  Constant : Constant  Value=overcurr_ctrl.i_lim
  Constant1 : Constant  Value=[0; 0]
  Constant2 : Constant  Value=[0;0]
  Logical Operator : Logic  Operator=OR  AllPortsSameDT=off  OutDataTypeStr=boolean
  NOT1 : Logic  Operator=NOT  IconShape=distinctive  AllPortsSameDT=off  OutDataTypeStr=boolean
  NOT2 : Logic  Operator=NOT  IconShape=distinctive  AllPortsSameDT=off  OutDataTypeStr=boolean
  PQCtrl : eeDiscretePi/Discrete PI Controller  Kp=overcurr_ctrl.kp  Ki=overcurr_ctrl.ki  Kaw=100  x0=0  Ts=-1
      settings: LibrarySourceBlock=ee_sl_lib/General Control/Discrete PI Controller
  Relational Operator : RelationalOperator  Operator=<=  OutDataTypeStr=boolean  RndMeth=Simplest  InputSameDT=off
  Relay : Relay  OnSwitchValue=0  OffSwitchValue=-0.03  OnOutputValue=0  OffOutputValue=1
  Sum : Sum  Inputs=|+-
  Sum1 : Sum  Inputs=++|
  Sum2 : Sum  Inputs=++|
  Sum3 : Sum  Inputs=|+-
  Switch : Switch  Criteria=u2 > Threshold  SaturateOnIntegerOverflow=off  InputSameDT=off
  Terminator : Terminator
  Terminator1 : Terminator
  abs : Subsystem
  m : Outport
  v_pcc_f : Outport  Port=2
  dm_corr : Outport  Port=3
  active : Outport  Port=4
  lambda : Outport  Port=5
  wires:
  i_ref/1 -> Sum/1
  feedforward/1 -> Sum1/1
  i/1 -> abs/1(x), Sum/2
  NOT1/1 -> Logical Operator/2
  Logical Operator/1 -> Switch/2, NOT2/1, PQCtrl/3
  Constant/1 -> Sum3/2
  enable/1 -> NOT1/1
  abs/1(abs) -> Sum3/1
  PQCtrl/1 -> dm_corr/1, Sum1/2  "i_ref_dq"
  Sum1/1 -> Sum2/2
  antiwind/1 -> PQCtrl/2
  Sum/1 -> Switch/3
  NOT2/1 -> active/1
  Constant1/1 -> Switch/1
  Switch/1 -> PQCtrl/1
  w/1 -> Terminator1/1
  v_pcc/1 -> Terminator/1
  Constant2/1 -> lambda/1
  v_pcc_lp/1 -> Sum2/1, v_pcc_f/1
  Sum2/1 -> m/1
  Sum3/1 -> Relay/1
  Relay/1 -> Logical Operator/1

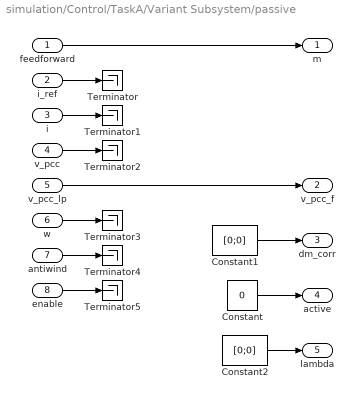
== system simulation/Control/TaskA/Variant Subsystem/passive ==
  feedforward : Inport
  i_ref : Inport  Port=2
  i : Inport  Port=3
  v_pcc : Inport  Port=4
  v_pcc_lp : Inport  Port=5
  w : Inport  Port=6
  antiwind : Inport  Port=7
  enable : Inport  Port=8
  Constant : Constant  Value=0
  Constant1 : Constant  Value=[0;0]
  Constant2 : Constant  Value=[0;0]
  Terminator{,1..5} (6 alike) : Terminator
  m : Outport
  v_pcc_f : Outport  Port=2
  dm_corr : Outport  Port=3
  active : Outport  Port=4
  lambda : Outport  Port=5
  wires:
  Constant/1 -> active/1
  feedforward/1 -> m/1
  i_ref/1 -> Terminator/1
  enable/1 -> Terminator5/1
  antiwind/1 -> Terminator4/1
  w/1 -> Terminator3/1
  v_pcc/1 -> Terminator2/1
  i/1 -> Terminator1/1
  v_pcc_lp/1 -> v_pcc_f/1
  Constant1/1 -> dm_corr/1
  Constant2/1 -> lambda/1

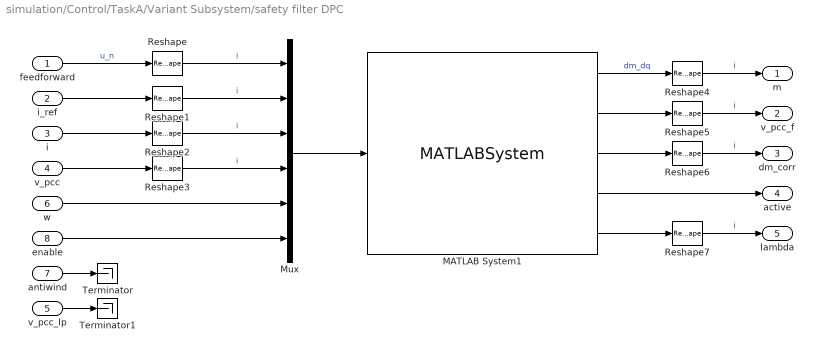
== system simulation/Control/TaskA/Variant Subsystem/safety filter DPC ==
  feedforward : Inport
  i_ref : Inport  Port=2
  i : Inport  Port=3
  v_pcc : Inport  Port=4
  v_pcc_lp : Inport  Port=5
  w : Inport  Port=6
  antiwind : Inport  Port=7
  enable : Inport  Port=8
  MATLAB System1 : MATLABSystem  System=SafetyFilterSystemDPC  ts=ctrl.ts  f_data=safety.f_data  G_data=safety.G_data  V_data=safety.V_data  B_data=safety.B_data  nV_data=safety.nV_data  nB_data=safety.nB_data  gamma_V_data=safety.gamma_V_data  gamma_B_data=safety.gamma_B_data  r=grid.r1  l=grid.l1  init_vpcc_f=[ctrl.init_vpeak; 0]  SimulateUsing=Code generation
      mask Type: SafetyFilterSystemDPC
      mask Display:
      | disp('SafetyFilterSystemDPC');
      | port_label('input',1,'u');
      | port_label('output',1,'m');
      | port_label('output',2,'dv_pcc_f');
      | port_label('output',3,'dm_corr');
      | port_label('output',4,'active');
      | port_label('output',5,'lambda');
  Mux : Mux  Inputs=[2 2 2 2 1 1]
  Reshape{,1..3} (4 alike) : Reshape  OutputDimensionality=Customize  OutputDimensions=[2,1]
  Reshape{4..7} (4 alike) : Reshape  OutputDimensionality=Customize  OutputDimensions=[2]
  Terminator : Terminator
  Terminator1 : Terminator
  m : Outport
  v_pcc_f : Outport  Port=2
  dm_corr : Outport  Port=3
  active : Outport  Port=4
  lambda : Outport  Port=5
  wires:
  MATLAB System1/4 -> active/1
  Reshape1/1 -> Mux/2  "i"
  i_ref/1 -> Reshape1/1
  Reshape3/1 -> Mux/4  "i"
  i/1 -> Reshape2/1
  feedforward/1 -> Reshape/1  "u_n"
  enable/1 -> Mux/6
  Mux/1 -> MATLAB System1/1
  w/1 -> Mux/5
  Reshape2/1 -> Mux/3  "i"
  Reshape4/1 -> m/1  "i"
  antiwind/1 -> Terminator/1
  v_pcc/1 -> Reshape3/1
  MATLAB System1/1 -> Reshape4/1  "dm_dq"
  Reshape/1 -> Mux/1  "i"
  MATLAB System1/5 -> Reshape7/1
  MATLAB System1/2 -> Reshape5/1
  MATLAB System1/3 -> Reshape6/1
  Reshape5/1 -> v_pcc_f/1  "i"
  Reshape6/1 -> dm_corr/1  "i"
  Reshape7/1 -> lambda/1  "i"
  v_pcc_lp/1 -> Terminator1/1

== system simulation/Control/TaskA/output lim/abs ==
  x : Inport
  Dot Product : DotProduct  OutDataTypeStr=Inherit: Inherit via internal rule
  Sqrt3 : Sqrt
  abs : Outport
  wires:
  Sqrt3/1 -> abs/1
  x/1 -> Dot Product/2, Dot Product/1
  Dot Product/1 -> Sqrt3/1

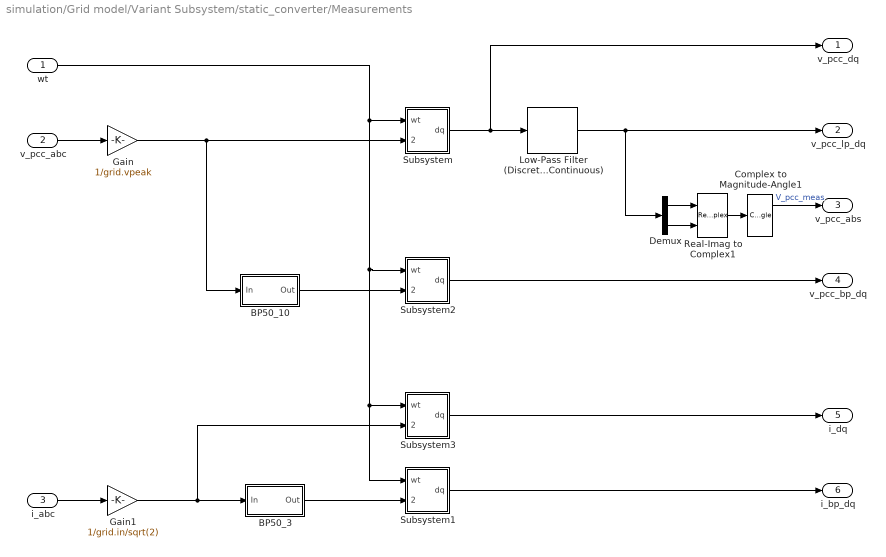
== system simulation/Grid model/Variant Subsystem/static_converter/Measurements ==
  wt : Inport
  v_pcc_abc : Inport  Port=2
  i_abc : Inport  Port=3
  BP50_10 : Subsystem  DialogController=fdesignblkfcn  InitFcn=fdesignblkfcn(gcbh, {'InitFcn'});  mask(Bandpass Filter){}
      mask help: dsp:DSPFilterDesignBlockDialog:BandpassFdesign_MaskDesc
      settings: CopyFcn=fdesignblkfcn(gcbh, {'CopyFcn'});
      mask Help: helpview(mapfilelocation('dsp'), 'dspbandpassfilter');
      mask Display: disp('Bandpass');
  BP50_3 : Subsystem  DialogController=fdesignblkfcn  InitFcn=fdesignblkfcn(gcbh, {'InitFcn'});  mask(Bandpass Filter){}
      mask help: dsp:DSPFilterDesignBlockDialog:BandpassFdesign_MaskDesc
      settings: CopyFcn=fdesignblkfcn(gcbh, {'CopyFcn'});
      mask Help: helpview(mapfilelocation('dsp'), 'dspbandpassfilter');
      mask Display: disp('Bandpass');
  Complex to Magnitude-Angle1 : ComplexToMagnitudeAngle
  Demux : Demux  Outputs=2
  Gain : Gain  Gain=1/grid.vpeak
  Gain1 : Gain  Gain=1/grid.in/sqrt(2)
  Low-Pass Filter (Discrete or Continuous) : eeGeneralControl/Low-Pass Filter (Discrete or Continuous)  K=1  T=10/grid.w0  B=inf  A=-inf  init_option=Inherited from block input  x0=0  Ts=-1
  Real-Imag to Complex1 : RealImagToComplex
  Subsystem : Subsystem
  Subsystem1 : Subsystem
  Subsystem2 : Subsystem
  Subsystem3 : Subsystem
  v_pcc_dq : Outport
  v_pcc_lp_dq : Outport  Port=2
  v_pcc_abs : Outport  Port=3
  v_pcc_bp_dq : Outport  Port=4
  i_dq : Outport  Port=5
  i_bp_dq : Outport  Port=6
  wires:
  v_pcc_abc/1 -> Gain/1
  Subsystem/1(dq) -> v_pcc_dq/1, Low-Pass Filter (Discrete or Continuous)/1
  Gain/1 -> BP50_10/1(In), Subsystem/2(abc)
  i_abc/1 -> Gain1/1
  BP50_3/1(Out) -> Subsystem1/2(abc)
  Subsystem1/1(dq) -> i_bp_dq/1
  Gain1/1 -> Subsystem3/2(abc), BP50_3/1(In)
  Low-Pass Filter (Discrete or Continuous)/1 -> Demux/1, v_pcc_lp_dq/1
  Real-Imag to Complex1/1 -> Complex to Magnitude-Angle1/1
  Demux/1 -> Real-Imag to Complex1/1
  Demux/2 -> Real-Imag to Complex1/2
  Complex to Magnitude-Angle1/1 -> v_pcc_abs/1  "V_pcc_meas"
  BP50_10/1(Out) -> Subsystem2/2(abc)
  Subsystem2/1(dq) -> v_pcc_bp_dq/1
  wt/1 -> Subsystem2/1(wt), Subsystem3/1(wt), Subsystem1/1(wt), Subsystem/1(wt)
  Subsystem3/1(dq) -> i_dq/1

== system simulation/Grid model/Variant Subsystem/static_converter/PLL1 ==
  v_pcc_dq : Inport
  enable : Inport  Port=2
  Complex to Magnitude-Angle : ComplexToMagnitudeAngle
  Constant : Constant  Value=0
  Constant1 : Constant  Value=0
  Demux6 : Demux  Outputs=2
  Discrete PI Controller : eeDiscretePi/Discrete PI Controller  Kp=pll.kp  Ki=pll.ki  Kaw=1  x0=1  Ts=-1
      settings: LibrarySourceBlock=ee_sl_lib/General Control/Discrete PI Controller
  Discrete-Time Integrator : DiscreteIntegrator  gainval=grid.w0  SampleTime=-1  ICPrevOutput=DiscIntNeverNeededParam  ICPrevScaledInput=DiscIntNeverNeededParam
  NOT1 : Logic  Operator=NOT  IconShape=distinctive  AllPortsSameDT=off  OutDataTypeStr=boolean
  Real-Imag to Complex : RealImagToComplex
  Switch : Switch  Criteria=u2 > Threshold  SaturateOnIntegerOverflow=off  InputSameDT=off
  Terminator7 : Terminator
  wt : Outport
  w : Outport  Port=2
  wires:
  v_pcc_dq/1 -> Demux6/1  "v_pcc_dq"
  Complex to Magnitude-Angle/1 -> Terminator7/1
  Demux6/2 -> Real-Imag to Complex/2  "v_pll_q"
  Complex to Magnitude-Angle/2 -> Switch/3  "theta_v_pll"
  Real-Imag to Complex/1 -> Complex to Magnitude-Angle/1
  Demux6/1 -> Real-Imag to Complex/1  "v_pll_d"
  Constant/1 -> Discrete PI Controller/2
  Discrete PI Controller/1 -> w/1, Discrete-Time Integrator/1
  Discrete-Time Integrator/1 -> wt/1
  NOT1/1 -> Switch/2, Discrete PI Controller/3
  enable/1 -> NOT1/1
  Switch/1 -> Discrete PI Controller/1
  Constant1/1 -> Switch/1

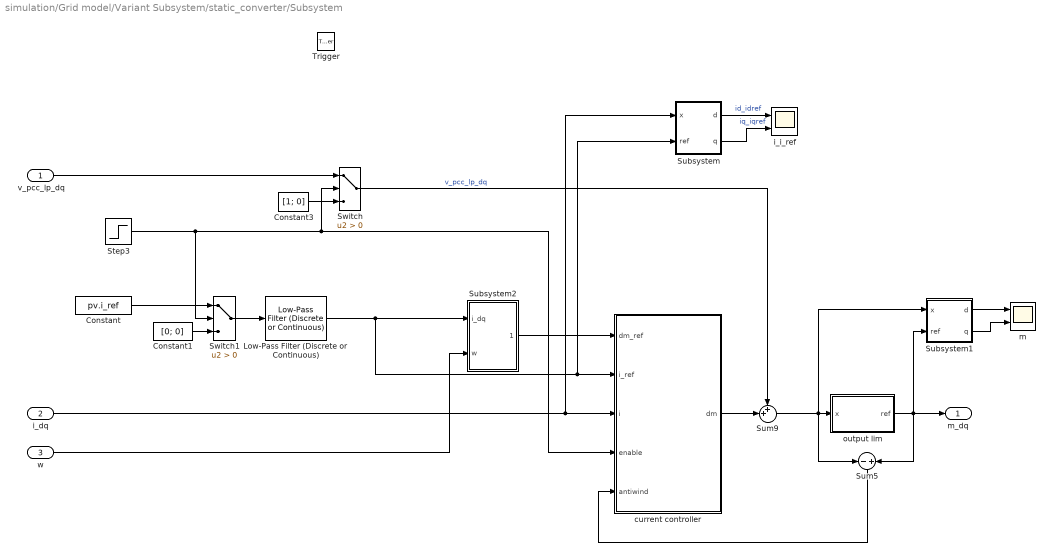
== system simulation/Grid model/Variant Subsystem/static_converter/Subsystem ==
  v_pcc_lp_dq : Inport
  i_dq : Inport  Port=2
  w : Inport  Port=3
  Trigger : TriggerPort  VariantControl=(inherit)
  Constant : Constant  Value=pv.i_ref
  Constant1 : Constant  Value=[0; 0]
  Constant3 : Constant  Value=[1; 0]
  Low-Pass Filter (Discrete or Continuous) : eeGeneralControl/Low-Pass Filter (Discrete or Continuous)  K=1  T=1e-2  B=inf  A=-inf  init_option=Inherited from block input  x0=0  Ts=-1
  Step3 : Step  Time=pv.ctrl_enable
  Subsystem : Subsystem
  Subsystem1 : Subsystem
  Subsystem2 : Subsystem
  Sum5 : Sum  Inputs=-|+
  Sum9 : Sum  Inputs=++|
  Switch : Switch  Criteria=u2 > Threshold  SaturateOnIntegerOverflow=off  InputSameDT=off
  Switch1 : Switch  Criteria=u2 > Threshold  SaturateOnIntegerOverflow=off  InputSameDT=off
  current controller : Subsystem  VariantControl=overcurr_ctrl.sel==1
  i_i_ref : Scope  NumInputPorts=2
  m : Scope  NumInputPorts=2
  output lim : Subsystem
  m_dq : Outport
  wires:
  i_dq/1 -> current controller/3(i), Subsystem/1(x)
  Switch/1 -> Sum9/1  "v_pcc_lp_dq"
  current controller/1(dm) -> Sum9/2
  Step3/1 -> Switch1/2, Switch/2, current controller/4(enable)
  Switch1/1 -> Low-Pass Filter (Discrete or Continuous)/1
  Sum9/1 -> output lim/1(x), Subsystem1/1(x), Sum5/1
  w/1 -> Subsystem2/2(w)
  v_pcc_lp_dq/1 -> Switch/1
  Constant3/1 -> Switch/3
  Sum5/1 -> current controller/5(antiwind)
  Subsystem/1(d) -> i_i_ref/1  "id_idref"
  Subsystem/2(q) -> i_i_ref/2  "iq_iqref"
  Subsystem1/2(q) -> m/2
  Subsystem1/1(d) -> m/1
  Low-Pass Filter (Discrete or Continuous)/1 -> Subsystem2/1(i_dq), current controller/2(i_ref), Subsystem/2(ref)
  Constant/1 -> Switch1/1
  Constant1/1 -> Switch1/3
  Subsystem2/1(dm_dq) -> current controller/1(dm_ref)
  output lim/1(ref) -> Subsystem1/2(ref), m_dq/1, Sum5/2

== system simulation/Control/TaskA/Variant Subsystem/current controller/abs ==
  x : Inport
  Dot Product : DotProduct  OutDataTypeStr=Inherit: Inherit via internal rule
  Sqrt3 : Sqrt
  abs : Outport
  wires:
  Sqrt3/1 -> abs/1
  x/1 -> Dot Product/2, Dot Product/1
  Dot Product/1 -> Sqrt3/1

== system simulation/Grid model/Variant Subsystem/static_converter/Measurements/BP50_10 ==
  In : Inport
  Generated Filter Block : dsparch4/Biquad Filter  Tag=BlockMethodSubSystem  FilterSource=Dialog parameters  CoeffSource=Specify via dialog  FilterObject=BQF  IIRFiltStruct=Direct form II  BiQuadCoeffs=[2 0 -2 1 -1.99996903213533184 0.99996913076816718]  ScaleValues=[4.98592317955378183e-08;154.7819266430281]  IC=0  ICnum=0  ICden=0  a0Flag=Warning  optimizeScaleValues=off  ScaleValueMode=Specify via input port (g)  roundingMode=Floor  overflowMode=off  scaleValueFracLength=14  denProdOutputFracLength=30  denAccumFracLength=30  secondMemoryFracLength=15
  Out : Outport  VectorParamsAs1DForOutWhenUnconnected=off
  wires:
  In/1 -> Generated Filter Block/1
  Generated Filter Block/1 -> Out/1

== system simulation/Grid model/Variant Subsystem/static_converter/Measurements/BP50_3 ==
  In : Inport
  Generated Filter Block : dsparch4/Biquad Filter  Tag=BlockMethodSubSystem  FilterSource=Dialog parameters  CoeffSource=Specify via dialog  FilterObject=BQF  IIRFiltStruct=Direct form II  BiQuadCoeffs=[2 0 -2 1 -1.99996903213533184 0.99996913076816718]  ScaleValues=[4.98592317955378183e-08;154.7819266430281]  IC=0  ICnum=0  ICden=0  a0Flag=Warning  optimizeScaleValues=off  ScaleValueMode=Specify via input port (g)  roundingMode=Floor  overflowMode=off  scaleValueFracLength=14  denProdOutputFracLength=30  denAccumFracLength=30  secondMemoryFracLength=15
  Out : Outport  VectorParamsAs1DForOutWhenUnconnected=off
  wires:
  In/1 -> Generated Filter Block/1
  Generated Filter Block/1 -> Out/1

== system simulation/Grid model/Variant Subsystem/static_converter/Measurements/Subsystem ==
  wt : Inport
  abc : Inport  Port=2
  Demux6 : Demux  Outputs=3
  Mux : Mux  Inputs=2
  Terminator7 : Terminator
  abc_dq_1 : spsabctodq0Lib/abc to dq0  Alignment=Aligned with phase A axis
  dq : Outport
  wires:
  Demux6/3 -> Terminator7/1
  Demux6/2 -> Mux/2  "v_pll_q"
  wt/1 -> abc_dq_1/2
  Mux/1 -> dq/1
  Demux6/1 -> Mux/1  "v_pll_d"
  abc/1 -> abc_dq_1/1
  abc_dq_1/1 -> Demux6/1

== system simulation/Grid model/Variant Subsystem/static_converter/Measurements/Subsystem1 ==
  wt : Inport
  abc : Inport  Port=2
  Demux6 : Demux  Outputs=3
  Mux : Mux  Inputs=2
  Terminator7 : Terminator
  abc_dq_1 : spsabctodq0Lib/abc to dq0  Alignment=Aligned with phase A axis
  dq : Outport
  wires:
  Demux6/3 -> Terminator7/1
  Demux6/2 -> Mux/2  "v_pll_q"
  wt/1 -> abc_dq_1/2
  Mux/1 -> dq/1
  Demux6/1 -> Mux/1  "v_pll_d"
  abc/1 -> abc_dq_1/1
  abc_dq_1/1 -> Demux6/1

== system simulation/Grid model/Variant Subsystem/static_converter/Measurements/Subsystem2 ==
  wt : Inport
  abc : Inport  Port=2
  Demux6 : Demux  Outputs=3
  Mux : Mux  Inputs=2
  Terminator7 : Terminator
  abc_dq_1 : spsabctodq0Lib/abc to dq0  Alignment=Aligned with phase A axis
  dq : Outport
  wires:
  Demux6/3 -> Terminator7/1
  Demux6/2 -> Mux/2  "v_pll_q"
  wt/1 -> abc_dq_1/2
  Mux/1 -> dq/1
  Demux6/1 -> Mux/1  "v_pll_d"
  abc/1 -> abc_dq_1/1
  abc_dq_1/1 -> Demux6/1

== system simulation/Grid model/Variant Subsystem/static_converter/Measurements/Subsystem3 ==
  wt : Inport
  abc : Inport  Port=2
  Demux6 : Demux  Outputs=3
  Mux : Mux  Inputs=2
  Terminator7 : Terminator
  abc_dq_1 : spsabctodq0Lib/abc to dq0  Alignment=Aligned with phase A axis
  dq : Outport
  wires:
  Demux6/3 -> Terminator7/1
  Demux6/2 -> Mux/2  "v_pll_q"
  wt/1 -> abc_dq_1/2
  Mux/1 -> dq/1
  Demux6/1 -> Mux/1  "v_pll_d"
  abc/1 -> abc_dq_1/1
  abc_dq_1/1 -> Demux6/1

== system simulation/Grid model/Variant Subsystem/static_converter/Subsystem/Subsystem ==
  x : Inport
  ref : Inport  Port=2
  Demux : Demux  Outputs=2
  Demux1 : Demux  Outputs=2
  Mux1 : Mux  Inputs=2
  Mux2 : Mux  Inputs=2
  d : Outport
  q : Outport  Port=2
  wires:
  Mux2/1 -> q/1
  ref/1 -> Demux1/1
  Demux/2 -> Mux2/1
  Demux1/2 -> Mux2/2
  Demux/1 -> Mux1/1
  Demux1/1 -> Mux1/2
  Mux1/1 -> d/1
  x/1 -> Demux/1

== system simulation/Grid model/Variant Subsystem/static_converter/Subsystem/Subsystem1 ==
  x : Inport
  ref : Inport  Port=2
  Demux : Demux  Outputs=2
  Demux1 : Demux  Outputs=2
  Mux1 : Mux  Inputs=2
  Mux2 : Mux  Inputs=2
  d : Outport
  q : Outport  Port=2
  wires:
  Mux2/1 -> q/1
  ref/1 -> Demux1/1
  Demux/2 -> Mux2/1
  Demux1/2 -> Mux2/2
  Demux/1 -> Mux1/1
  Demux1/1 -> Mux1/2
  Mux1/1 -> d/1
  x/1 -> Demux/1

== system simulation/Grid model/Variant Subsystem/static_converter/Subsystem/Subsystem2 ==
  i_dq : Inport
  w : Inport  Port=2
  Gain : Gain  Gain=J  Multiplication=Matrix(K*u) (u vector)
  Gain1 : Gain  Gain=ctrl.l1
  Gain2 : Gain  Gain=ctrl.r1
  Product : Product
  Sum8 : Sum  Inputs=++|
  dm_dq : Outport
  wires:
  Gain1/1 -> Sum8/2
  Sum8/1 -> dm_dq/1  "dm_dq"
  Product/1 -> Gain/1
  Gain/1 -> Gain1/1  "dm_dq"
  w/1 -> Product/1
  i_dq/1 -> Gain2/1, Product/2
  Gain2/1 -> Sum8/1

== system simulation/Grid model/Variant Subsystem/static_converter/Subsystem/current controller ==
  dm_ref : Inport
  i_ref : Inport  Port=2
  i : Inport  Port=3
  enable : Inport  Port=4
  antiwind : Inport  Port=5
  Constant1 : Constant  Value=[0; 0]
  NOT1 : Logic  Operator=NOT  IconShape=distinctive  AllPortsSameDT=off  OutDataTypeStr=boolean
  PQCtrl : eeDiscretePi/Discrete PI Controller  Kp=overcurr_ctrl.kp  Ki=overcurr_ctrl.ki  Kaw=1  x0=0  Ts=-1
      settings: LibrarySourceBlock=ee_sl_lib/General Control/Discrete PI Controller
  Sum : Sum  Inputs=|+-
  Sum1 : Sum  Inputs=++|
  Switch : Switch  Criteria=u2 > Threshold  SaturateOnIntegerOverflow=off  InputSameDT=off
  dm : Outport
  wires:
  i_ref/1 -> Sum/1
  dm_ref/1 -> Sum1/1
  i/1 -> Sum/2
  enable/1 -> NOT1/1
  PQCtrl/1 -> Sum1/2  "i_ref_dq"
  Sum1/1 -> dm/1
  antiwind/1 -> PQCtrl/2
  Sum/1 -> Switch/3
  NOT1/1 -> Switch/2, PQCtrl/3
  Constant1/1 -> Switch/1
  Switch/1 -> PQCtrl/1

== system simulation/Grid model/Variant Subsystem/static_converter/Subsystem/output lim ==
  x : Inport
  Constant6 : Constant  Value=soa.m_max
  Divide1 : Product  Inputs=*/
  Product4 : Product
  abs : Subsystem
  m_c_max<=u : Saturate  UpperLimit=inf  LowerLimit=soa.m_max
  ref : Outport
  wires:
  abs/1(abs) -> m_c_max<=u/1
  Constant6/1 -> Divide1/1
  Divide1/1 -> Product4/2  "a_s"
  m_c_max<=u/1 -> Divide1/2
  x/1 -> abs/1(x), Product4/1
  Product4/1 -> ref/1

== system simulation/Grid model/Variant Subsystem/static_converter/Subsystem/output lim/abs ==
  x : Inport
  Dot Product : DotProduct  OutDataTypeStr=Inherit: Inherit via internal rule
  Sqrt3 : Sqrt
  abs : Outport
  wires:
  Sqrt3/1 -> abs/1
  x/1 -> Dot Product/2, Dot Product/1
  Dot Product/1 -> Sqrt3/1
